simulink model "PurePursuit_Tractor_Home"  (R2025b)
settings: Solver=FixedStepDiscrete  StartTime=0.0  StopTime=tmax  FixedStep=1/120  RelTol=1e-3
values from neighbouring files (symbols this model uses):
  Ts = 1./fs    (= 0.00833333333333)    [TruckLab_A2_Home.m]    (also in TruckLab_A2_Lab.m)
undefined symbols (not defined in the file or in its folder): controller, DiscIntNeverNeededParam, p, path
settings Model: Creator=jakub  LastModifiedBy=20224886
settings SolverCC: AlgebraicLoopSolver=TrustRegion
settings OptimizationCC: DefaultParameterBehavior=Inlined  EnhancedBackFolding=on  PassReuseOutputArgsAs=Individual arguments  ZeroExternalMemoryAtStartup=off  ZeroInternalMemoryAtStartup=off  MaxStackSize=64  OptimizeBlockOrder=speed  DifferentSizesBufferReuse=on  OptimizationCustomize=off  EfficientTunableParamExpr=on
settings DebuggingCC: ParameterTunabilityLossMsg=error  UnconnectedInputMsg=warning  UnconnectedOutputMsg=warning  UnconnectedLineMsg=warning
settings HardwareCC: ProdBitPerPointer=32.0  ProdBitPerSizeT=32.0  ProdBitPerPtrDiffT=32.0  ProdLargestAtomicFloat=None  ProdIntDivRoundTo=Undefined  ProdEndianess=Unspecified  ProdWordSize=32.0  ProdHWDeviceType=Generic->Unspecified (assume 32-bit Generic)  UseEmbeddedCoderFeatures=off
settings ModelReferenceCC: EnableRefExpFcnMdlSchedulingChecks=on
settings SFSimCC: MATLABDynamicMemAlloc=off
settings RTWCC: SystemTargetFile=ert.tlc  HardwareBoard=Robot Operating System (ROS)  TLCOptions="-aInlineSetEventsForThisBaseRateFcn=TLC_FALSE -aSuppressMultiTaskScheduler=TLC_FALSE  -aRateBasedStepFcn=0"  TemplateMakefile=ert_default_tmf  Toolchain=Catkin  TargetLang=C++  GPUComputeCapability=3.5  Description=Embedded Coder
settings CodeAppCC: ForceParamTrailComments=on  IgnoreCustomStorageClasses=off  OperatorAnnotations=on  SimulinkDataObjDesc=on  SFDataObjDesc=on  InsertBlockDesc=on
settings ERTTargetCC: SupportNonInlinedSFcns=on

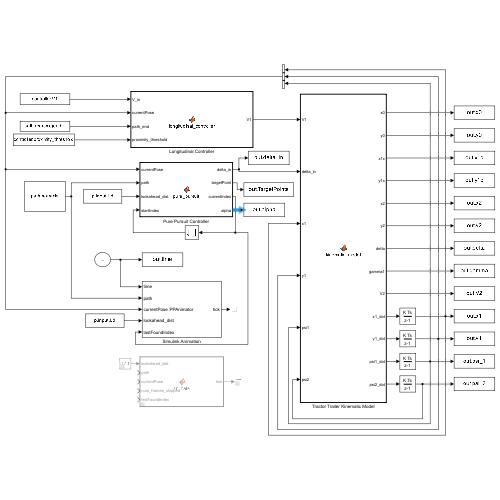
[thumbnail: Simulink's stored preview of the top-level diagram]
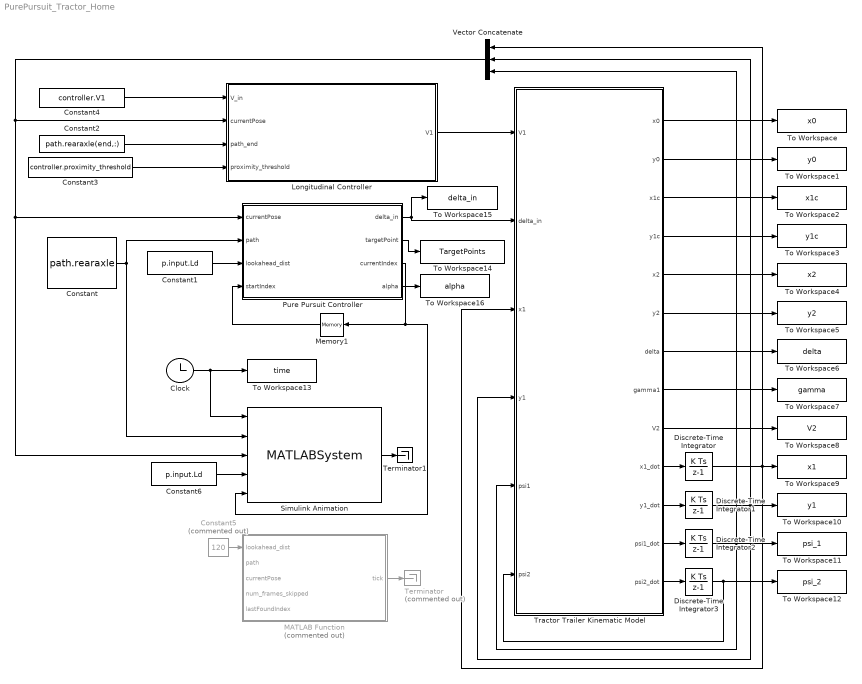
== system PurePursuit_Tractor_Home ==
  Clock : Clock
  Constant : Constant  Value=path.rearaxle
  Constant1 : Constant  Value=p.input.Ld
  Constant2 : Constant  Value=path.rearaxle(end,:)
  Constant3 : Constant  Value=controller.proximity_threshold
  Constant4 : Constant  Value=controller.V1
  Constant5 : Constant  Commented=on  Value=120
  Constant6 : Constant  Value=p.input.Ld
  Discrete-Time Integrator : DiscreteIntegrator  InitialCondition=p.init.x10  SampleTime=Ts  ICPrevOutput=DiscIntNeverNeededParam  ICPrevScaledInput=DiscIntNeverNeededParam
  Discrete-Time Integrator1 : DiscreteIntegrator  InitialCondition=p.init.y10  SampleTime=Ts  ICPrevOutput=DiscIntNeverNeededParam  ICPrevScaledInput=DiscIntNeverNeededParam
  Discrete-Time Integrator2 : DiscreteIntegrator  InitialCondition=p.init.psi10  SampleTime=Ts  ICPrevOutput=DiscIntNeverNeededParam  ICPrevScaledInput=DiscIntNeverNeededParam
  Discrete-Time Integrator3 : DiscreteIntegrator  InitialCondition=p.init.psi20  SampleTime=Ts  ICPrevOutput=DiscIntNeverNeededParam  ICPrevScaledInput=DiscIntNeverNeededParam
  Longitudinal Controller : MATLAB Function  TreatAsAtomicUnit=on
  MATLAB Function : MATLAB Function  Commented=on  TreatAsAtomicUnit=on
  Memory1 : Memory  InitialCondition=1  InheritSampleTime=on
  Pure Pursuit Controller : MATLAB Function  TreatAsAtomicUnit=on
  Simulink Animation : MATLABSystem  System=PPAnimator  desiredFrameRate=5  simStepSize=1  SimulateUsing=Interpreted execution
      mask Type: PPAnimator
  Terminator : Terminator  Commented=on
  Terminator1 : Terminator
  To Workspace : ToWorkspace  VariableName=x0  SaveFormat=Timeseries  SampleTime=-1
  To Workspace1 : ToWorkspace  VariableName=y0  SaveFormat=Timeseries  SampleTime=-1
  To Workspace10 : ToWorkspace  VariableName=y1  SaveFormat=Timeseries  SampleTime=-1
  To Workspace11 : ToWorkspace  VariableName=psi_1  SaveFormat=Timeseries  SampleTime=-1
  To Workspace12 : ToWorkspace  VariableName=psi_2  SaveFormat=Timeseries  SampleTime=-1
  To Workspace13 : ToWorkspace  VariableName=time  SaveFormat=Timeseries  SampleTime=-1
  To Workspace14 : ToWorkspace  VariableName=TargetPoints  SampleTime=Ts
      settings: Save2DSignal=2-D array (concatenate along first dimension)
  To Workspace15 : ToWorkspace  VariableName=delta_in  SaveFormat=Timeseries  SampleTime=-1
  To Workspace16 : ToWorkspace  VariableName=alpha  SaveFormat=Timeseries  SampleTime=-1
  To Workspace2 : ToWorkspace  VariableName=x1c  SaveFormat=Timeseries  SampleTime=-1
  To Workspace3 : ToWorkspace  VariableName=y1c  SaveFormat=Timeseries  SampleTime=-1
  To Workspace4 : ToWorkspace  VariableName=x2  SaveFormat=Timeseries  SampleTime=-1
  To Workspace5 : ToWorkspace  VariableName=y2  SaveFormat=Timeseries  SampleTime=-1
  To Workspace6 : ToWorkspace  VariableName=delta  SaveFormat=Timeseries  SampleTime=-1
  To Workspace7 : ToWorkspace  VariableName=gamma  SaveFormat=Timeseries  SampleTime=-1
  To Workspace8 : ToWorkspace  VariableName=V2  SaveFormat=Timeseries  SampleTime=-1
  To Workspace9 : ToWorkspace  VariableName=x1  SaveFormat=Timeseries  SampleTime=-1
  Tractor Trailer Kinematic Model : MATLAB Function  TreatAsAtomicUnit=on
  Vector Concatenate : Concatenate  NumInputs=3
  wires:
  Discrete-Time Integrator/1 -> Vector Concatenate/1, Tractor Trailer Kinematic Model/3(x1), To Workspace9/1
  Discrete-Time Integrator1/1 -> Vector Concatenate/2, To Workspace10/1, Tractor Trailer Kinematic Model/4(y1)
  Discrete-Time Integrator2/1 -> Tractor Trailer Kinematic Model/5(psi1), Vector Concatenate/3, To Workspace11/1
  Discrete-Time Integrator3/1 -> To Workspace12/1, Tractor Trailer Kinematic Model/6(psi2)
  Tractor Trailer Kinematic Model/9(V2) -> To Workspace8/1
  Tractor Trailer Kinematic Model/8(gamma1) -> To Workspace7/1
  Tractor Trailer Kinematic Model/6(y2) -> To Workspace5/1
  Tractor Trailer Kinematic Model/5(x2) -> To Workspace4/1
  Tractor Trailer Kinematic Model/4(y1c) -> To Workspace3/1
  Tractor Trailer Kinematic Model/3(x1c) -> To Workspace2/1
  Tractor Trailer Kinematic Model/2(y0) -> To Workspace1/1
  Tractor Trailer Kinematic Model/1(x0) -> To Workspace/1
  Clock/1 -> Simulink Animation/1, To Workspace13/1
  Tractor Trailer Kinematic Model/7(delta) -> To Workspace6/1
  Constant/1 -> Simulink Animation/2, Pure Pursuit Controller/2(path)
  Pure Pursuit Controller/3(currentIndex) -> Simulink Animation/5, Memory1/1
  Memory1/1 -> Pure Pursuit Controller/4(startIndex)
  Vector Concatenate/1 -> Longitudinal Controller/2(currentPose), Simulink Animation/3, Pure Pursuit Controller/1(currentPose)
  Constant2/1 -> Longitudinal Controller/3(path_end)
  Pure Pursuit Controller/2(targetPoint) -> To Workspace14/1
  Constant3/1 -> Longitudinal Controller/4(proximity_threshold)
  Tractor Trailer Kinematic Model/10(x1_dot) -> Discrete-Time Integrator/1
  Tractor Trailer Kinematic Model/13(psi2_dot) -> Discrete-Time Integrator3/1
  Tractor Trailer Kinematic Model/12(psi1_dot) -> Discrete-Time Integrator2/1
  Tractor Trailer Kinematic Model/11(y1_dot) -> Discrete-Time Integrator1/1
  Constant4/1 -> Longitudinal Controller/1(V_in)
  Longitudinal Controller/1(V1) -> Tractor Trailer Kinematic Model/1(V1)
  Pure Pursuit Controller/1(delta_in) -> Tractor Trailer Kinematic Model/2(delta_in), To Workspace15/1
  MATLAB Function/1(tick) -> Terminator/1
  Constant1/1 -> Pure Pursuit Controller/3(lookahead_dist)
  Constant5/1 -> MATLAB Function/1(lookahead_dist)
  Simulink Animation/1 -> Terminator1/1
  Constant6/1 -> Simulink Animation/4
  Pure Pursuit Controller/4(alpha) -> To Workspace16/1

== matlab function PurePursuit_Tractor_Home/Pure Pursuit Controller ==
  data: currentPose input; delta_in output; targetPoint output; path input; lookahead_dist input; startIndex input; currentIndex output; alpha output
function [delta_in,  targetPoint, currentIndex, alpha] = pure_pursuit(currentPose, path, lookahead_dist, startIndex)
%#codegen
% Inputs:
%   currentPose : [1x3] [x y psi]
%   path        : [N x 2] waypoints (fixed-size)
%   startIndex  : scalar segment index (1..N-1)
% Outputs:
%   delta_in    : scalar steering [rad]
%   currentIndex: scalar updated lastFoundIndex

targetPoint = [NaN, NaN];

% Tunables (make mask params or Simulink.Parameters if desired)
L1 = 0.263;                 % wheelbase [m]
delta_max = 38 *pi/180;     % max steering angle [rad]

x1 = currentPose(1); y1 = currentPose(2); psi1 = currentPose(3);

% ---- Step 1: target + index ----


% ---- Step 2: target direction alpha (atan2 + wrap) ----


% ---- Step 3: steering ----

== matlab function PurePursuit_Tractor_Home/Tractor Trailer Kinematic Model ==
  data: V1 input; x0 output; delta_in input; x1 input; y1 input; psi1 input; psi2 input; y0 output; x1c output; y1c output; x2 output; y2 output; delta output; gamma1 output; V2 output; x1_dot output; y1_dot output; psi1_dot output; psi2_dot output
function [x0,y0,x1c,y1c,x2,y2,delta,gamma1,V2,x1_dot,y1_dot,psi1_dot,psi2_dot]= kinematic_model(V1,delta_in,x1,y1,psi1, psi2)

L1=0.28;                          %wheel base of truck
L1c=0.055;                        % distance rear truck axle to first kingpin (positive means behind the axle)
L2=0.56;
delta_max =  38*pi/180;           % maximum steering angle front wheel [rad]
% gamma_max = 110*pi/180;           % maximum articulation angle [rad]

% % limit maximum steering angle within mechanical limits (hard stops)
delta    = max(-delta_max, min(delta_max,delta_in));  

% calculate the articulation angle (angle between tractor and semitrailer)
gamma1   = psi1 - psi2;

% front axle position
x0       = x1 + L1*cos(psi1);
y0       = y1 + L1*sin(psi1);

% 5th wheel tractor (coupling to semi-trailer) position
x1c      = x1 + L1c*cos(psi1);
y1c      = y1 + L1c*sin(psi1);

% semitrailer center axle position
x2       = x1c - L2*cos(psi2);
y2       = y1c - L2*sin(psi2);

% tractor dynamics
x1_dot   =  V1*cos(psi1);
y1_dot   =  V1*sin(psi1);
psi1_dot = (V1/L1)*tan(delta);

%semitrailer dynamics
V2       =   V1*cos(gamma1) - psi1_dot*L1c*sin(gamma1);
psi2_dot = ( V1*sin(gamma1) + psi1_dot*L1c*cos(gamma1) )/L2;

end

== matlab function PurePursuit_Tractor_Home/Longitudinal Controller ==
  data: V_in input; currentPose input size=3; V1 output; path_end input; proximity_threshold input
function V1 = longitudinal_controller(V_in, currentPose, path_end, proximity_threshold)
    % ---- STOPING CRITERION ----
    if euclidean_distance([currentPose(1), currentPose(2)], path_end) < proximity_threshold
        V1 = 0;
%         disp('STOP TRIGGERED');
    else
        V1 = V_in;
    end
    
% ================= Subfunctions =================
function d = euclidean_distance(p, q)
    dx = p(1) - q(1); 
    dy = p(2) - q(2);
    d  = sqrt(dx*dx + dy*dy);

== matlab function PurePursuit_Tractor_Home/MATLAB Function ==
  data: lookahead_dist input; path input; tick output; currentPose input; num_frames_skipped input; lastFoundIndex input
function tick = animate(lookahead_dist, path, currentPose, num_frames_skipped, lastFoundIndex)
%#codegen
coder.extrinsic('helpers.pure_pursuit_animation');

persistent n
if isempty(n); n = uint32(0); end
n = n + 1;

if n >= uint32(num_frames_skipped)
    n = uint32(0);
    % Call extrinsic animator at a reduced rate
    helpers.pure_pursuit_animation(path, currentPose, lookahead_dist, lastFoundIndex);
end

% Dummy scalar output keeps the block valid
tick = uint8(0);
